simulink model "Crane3D_first_lqr"  (R2015a)
settings: Solver=ode5  SolverMode=SingleTasking  StartTime=0.0  StopTime=30  FixedStep=T0  RelTol=1e-3  AbsTol=1e-6
values from neighbouring files (symbols this model uses):
  Al = [0  1     0 0 ... (first row only)    [req_lqr.m]
  Bl = [0; Km/T; 0; K*Km*omega^2/T]    [req_lqr.m]
  Cl = [1 0 0 0 ... (first row only)    [req_lqr.m]
  Klqr = lqr(Al,Bl,Q,R)    [req_lqr.m]
  L = transpose(place(transpose(Al),transpose(Cl), [-11 -10 -9 -11]))    [req_lqr.m]
  X0 = [0 0 0 0]    [req_lqr.m]
undefined symbols (not defined in the file or in its folder): Crane3D_RangeBit, Crane3D_ScaleCoeff
undefined symbols (not defined in the file): RTDAC4PCIBaseAddress, T0
settings Model: SimulationMode=external  CovSFcnEnable=off  ExtModeTrigDuration=100000  Creator=jims  LastModifiedBy=Student
settings DataIOCC: ExternalInput=[]  InitialState=[]  LimitDataPoints=off  MaxDataPoints=5000  SignalLoggingSaveFormat=ModelDataLogs  SaveOutput=off  SaveTime=off
settings OptimizationCC: BooleanDataType=off  OptimizeBlockIOStorage=off  BufferReuse=off  GlobalBufferReuse=off  ExpressionFolding=off  ExpressionDepthLimit=2147483647  LocalBlockOutputs=off  InitFltsAndDblsToZero=on
settings DebuggingCC: SaveWithParameterizedLinksMsg=none  UnderspecifiedInitializationDetection=Classic  MergeDetectMultiDrivingBlocksExec=none  SignalResolutionControl=TryResolveAllWithWarning  MultiTaskDSMMsg=warning  MultiTaskCondExecSysMsg=none  IntegerOverflowMsg=none  FcnCallInpInsideContextMsg=UseLocalSettings  StateNameClashWarn=warning  IntegerSaturationMsg=none
settings HardwareCC: ProdBitPerLong=64  ProdBitPerPointer=64  ProdIntDivRoundTo=Zero  ProdEndianess=LittleEndian  ProdWordSize=64  ProdHWDeviceType=Intel->x86-64  TargetBitPerLong=64  TargetBitPerPointer=64  TargetIntDivRoundTo=Zero  TargetEndianess=LittleEndian  TargetWordSize=64  TargetHWDeviceType=Intel->x86-64
settings RTWCC: SystemTargetFile=rtwin.tlc  TemplateMakefile=rtwin.tmf  Description=Real-Time Windows Target
settings RTWinTargetCC: TargetFcnLib=ansi_tfl_tmw.mat  TargetPreCompLibLocation=C:\Program Files\MATLAB\R2015aSP1\toolbox\sldrt\lib\win64  ModelReferenceCompliant=off  CompOptLevelCompliant=off

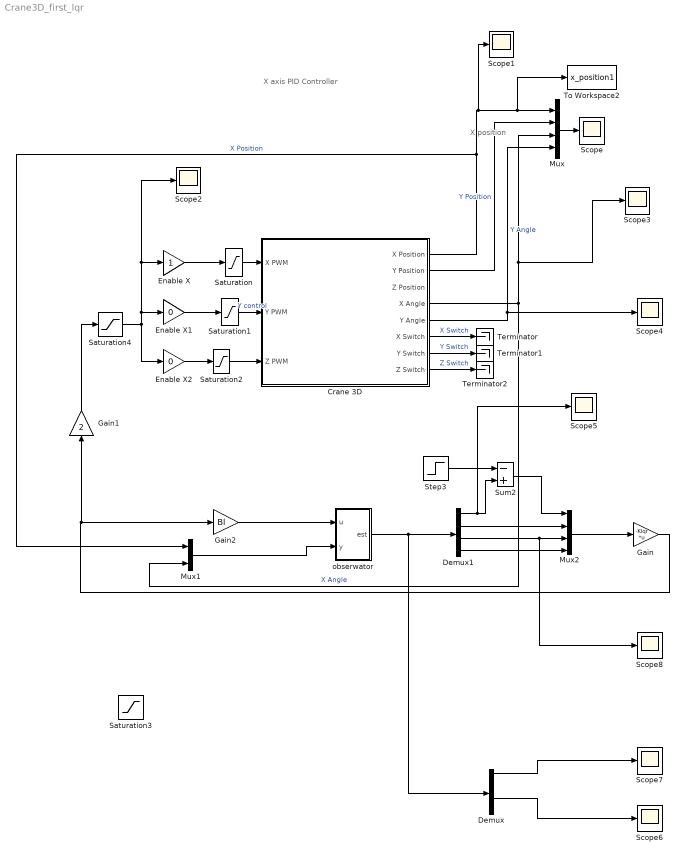
== system Crane3D_first_lqr ==
  note: X axis PID Controller
  note: X position
  Crane 3D : Subsystem  mask{BaseAddress=RTDAC4PCIBaseAddress, T0=T0}
      mask prompts: BaseAddress "Base Address:"; T0 "Sampling Period:"
      mask Display: image(imread('crane.jpeg'))
  Demux : Demux
  Demux1 : Demux
  Enable X : Gain  SaturateOnIntegerOverflow=on  OutDataTypeStr=Inherit: Same as input  ParamDataTypeStr=Inherit: Same as input
  Enable X1 : Gain  Gain=0  SaturateOnIntegerOverflow=on  OutDataTypeStr=Inherit: Same as input  ParamDataTypeStr=Inherit: Same as input
  Enable X2 : Gain  Gain=0  SaturateOnIntegerOverflow=on  OutDataTypeStr=Inherit: Same as input  ParamDataTypeStr=Inherit: Same as input
  Gain : Gain  Gain=-Klqr  Multiplication=Matrix(K*u) (u vector)
  Gain1 : Gain  Gain=2
  Gain2 : Gain  Gain=Bl
  Mux : Mux
  Mux1 : Mux  Inputs=2
  Mux2 : Mux
  Saturation{,1..4} (5 alike) : Saturate  UpperLimit=1  LowerLimit=-1
  Scope{,1..8} (9 alike) : Scope
      Scope settings: YMin=-0.25  YMax=4  SaveName=wsp
      Scope1 settings: YMin=1.38778e-17  YMax=0.35  SaveName=wsp1
      Scope2 settings: YMin=-0.1  YMax=0.65  SaveName=sterowanie
      Scope3 settings: YMin=-0.01  YMax=0.05  SaveName=wsp3
      Scope4 settings: YMin=-0.3  YMax=0.3  SaveName=wsp2
      Scope5 settings: YMin=0  YMax=0.12  SaveName=ScopeData2
      Scope6 settings: YMin=0.0881  YMax=0.088425
      Scope7 settings: YMin=0.27125  YMax=0.274
      Scope8 settings: YMin=-0.4  YMax=0.2  SaveName=ScopeData3
  Step3 : Step  Before=0.1  After=0.3  SampleTime=0
  Sum2 : Sum  Inputs=-+
  Terminator : Terminator
  Terminator1 : Terminator
  Terminator2 : Terminator
  To Workspace2 : ToWorkspace  VariableName=x_position1  SampleTime=-1
  "obserwator " : Subsystem
  wires:
  Crane 3D/6(X Switch) -> Terminator/1  "X Switch"
  Crane 3D/7(Y Switch) -> Terminator1/1  "Y Switch"
  Crane 3D/8(Z Switch) -> Terminator2/1  "Z Switch"
  Enable X/1 -> Saturation/1
  Crane 3D/4(X Angle) -> Mux/3, Scope3/1, Mux1/2  "X Angle"
  Crane 3D/5(Y Angle) -> Mux/4, Scope4/1  "Y Angle"
  Crane 3D/1(X Position) -> Mux1/1, Scope1/1, To Workspace2/1, Mux/1  "X Position"
  Saturation2/1 -> Crane 3D/3(Z PWM)
  Saturation1/1 -> Crane 3D/2(Y PWM)  "Y control"
  Saturation/1 -> Crane 3D/1(X PWM)
  Mux/1 -> Scope/1
  Crane 3D/2(Y Position) -> Mux/2  "Y Position"
  Enable X1/1 -> Saturation1/1
  Enable X2/1 -> Saturation2/1
  "obserwator "/1(est) -> Demux/1, Demux1/1
  Demux/3 -> Scope6/1
  Demux/1 -> Scope7/1
  Step3/1 -> Sum2/1
  Demux1/1 -> Scope5/1, Sum2/2
  Mux2/1 -> Gain/1
  Sum2/1 -> Mux2/1
  Demux1/2 -> Mux2/2
  Demux1/3 -> Scope8/1, Mux2/3
  Demux1/4 -> Mux2/4
  Saturation4/1 -> Enable X1/1, Scope2/1, Enable X/1, Enable X2/1
  Gain2/1 -> "obserwator "/1(u)
  Mux1/1 -> "obserwator "/2(y)
  Gain/1 -> Gain2/1, Gain1/1
  Gain1/1 -> Saturation4/1

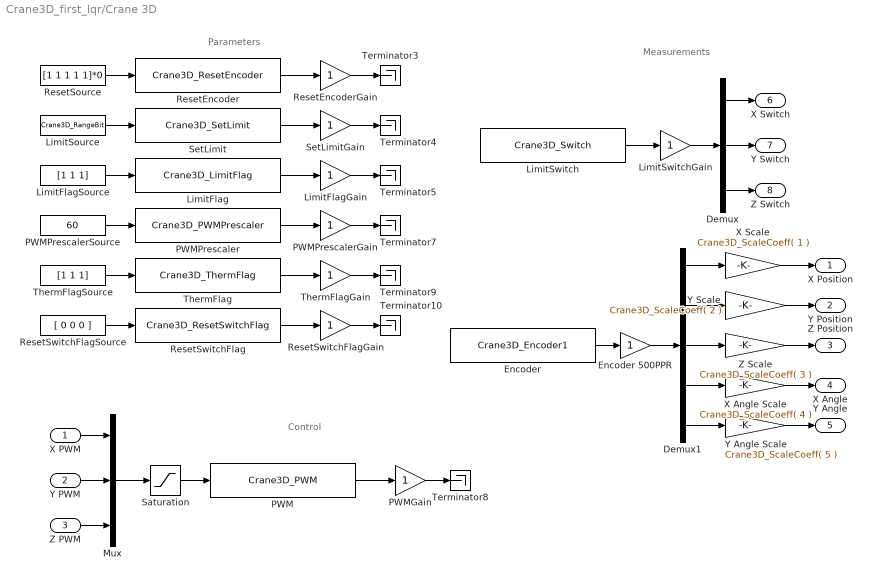
== system Crane3D_first_lqr/Crane 3D ==
  note: Parameters
  note: Control
  note: Measurements
  X PWM : Inport
  Y PWM : Inport  Port=2
  Z PWM : Inport  Port=3
  Demux : Demux  Outputs=3
  Demux1 : Demux  Outputs=5
  Encoder : S-Function  FunctionName=Crane3D_Encoder1  Parameters=BaseAddress, T0
  Encoder 500PPR : Gain  SaturateOnIntegerOverflow=on  OutDataTypeStr=Inherit: Same as input  ParamDataTypeStr=Inherit: Same as input
  LimitFlag : S-Function  FunctionName=Crane3D_LimitFlag  Parameters=BaseAddress, T0
  LimitFlagGain : Gain  SaturateOnIntegerOverflow=on  OutDataTypeStr=Inherit: Same as input  ParamDataTypeStr=Inherit: Same as input
  LimitFlagSource : Constant  Value=[1 1 1]
  LimitSource : Constant  Value=Crane3D_RangeBit
  LimitSwitch : S-Function  FunctionName=Crane3D_Switch  Parameters=BaseAddress, T0
  LimitSwitchGain : Gain  SaturateOnIntegerOverflow=on  OutDataTypeStr=Inherit: Same as input  ParamDataTypeStr=Inherit: Same as input
  Mux : Mux  Inputs=3
  PWM : S-Function  FunctionName=Crane3D_PWM  Parameters=BaseAddress, T0
  PWMGain : Gain  SaturateOnIntegerOverflow=on  OutDataTypeStr=Inherit: Same as input  ParamDataTypeStr=Inherit: Same as input
  PWMPrescaler : S-Function  FunctionName=Crane3D_PWMPrescaler  Parameters=BaseAddress, T0
  PWMPrescalerGain : Gain  SaturateOnIntegerOverflow=on  OutDataTypeStr=Inherit: Same as input  ParamDataTypeStr=Inherit: Same as input
  PWMPrescalerSource : Constant  Value=60
  ResetEncoder : S-Function  FunctionName=Crane3D_ResetEncoder  Parameters=BaseAddress, T0
  ResetEncoderGain : Gain  SaturateOnIntegerOverflow=on  OutDataTypeStr=Inherit: Same as input  ParamDataTypeStr=Inherit: Same as input
  ResetSource : Constant  Value=[1 1 1 1 1]*0
  "ResetSwitchFlag " : S-Function  FunctionName=Crane3D_ResetSwitchFlag  Parameters=BaseAddress, T0
  ResetSwitchFlagGain : Gain  SaturateOnIntegerOverflow=on  OutDataTypeStr=Inherit: Same as input  ParamDataTypeStr=Inherit: Same as input
  ResetSwitchFlagSource : Constant  Value=[ 0 0 0 ]
  Saturation : Saturate  UpperLimit=1  LowerLimit=-1
  SetLimit : S-Function  FunctionName=Crane3D_SetLimit  Parameters=BaseAddress, T0
  SetLimitGain : Gain  SaturateOnIntegerOverflow=on  OutDataTypeStr=Inherit: Same as input  ParamDataTypeStr=Inherit: Same as input
  Terminator{3..5,7..10} (7 alike) : Terminator
  "ThermFlag " : S-Function  FunctionName=Crane3D_ThermFlag  Parameters=BaseAddress, T0
  ThermFlagGain : Gain  SaturateOnIntegerOverflow=on  OutDataTypeStr=Inherit: Same as input  ParamDataTypeStr=Inherit: Same as input
  ThermFlagSource : Constant  Value=[1 1 1]
  X Angle Scale : Gain  Gain=Crane3D_ScaleCoeff( 4 )  OutDataTypeStr=Inherit: Same as input  ParamDataTypeStr=Inherit: Same as input
  X Scale : Gain  Gain=Crane3D_ScaleCoeff( 1 )  OutDataTypeStr=Inherit: Same as input  ParamDataTypeStr=Inherit: Same as input
  Y Angle Scale : Gain  Gain=Crane3D_ScaleCoeff( 5 )  OutDataTypeStr=Inherit: Same as input  ParamDataTypeStr=Inherit: Same as input
  Y Scale : Gain  Gain=Crane3D_ScaleCoeff( 2 )  OutDataTypeStr=Inherit: Same as input  ParamDataTypeStr=Inherit: Same as input
  Z Scale : Gain  Gain=Crane3D_ScaleCoeff( 3 )  OutDataTypeStr=Inherit: Same as input  ParamDataTypeStr=Inherit: Same as input
  X Position : Outport  InitialOutput=0
  Y Position : Outport  Port=2  InitialOutput=0
  Z Position : Outport  Port=3  InitialOutput=0
  X Angle : Outport  Port=4  InitialOutput=0
  Y Angle : Outport  Port=5  InitialOutput=0
  X Switch : Outport  Port=6  InitialOutput=0
  Y Switch : Outport  Port=7  InitialOutput=0
  Z Switch : Outport  Port=8  InitialOutput=0
  wires:
  Encoder 500PPR/1 -> Demux1/1
  Encoder/1 -> Encoder 500PPR/1
  Saturation/1 -> PWM/1
  Mux/1 -> Saturation/1
  PWM/1 -> PWMGain/1
  PWMGain/1 -> Terminator8/1
  ResetEncoder/1 -> ResetEncoderGain/1
  SetLimit/1 -> SetLimitGain/1
  LimitFlag/1 -> LimitFlagGain/1
  PWMPrescaler/1 -> PWMPrescalerGain/1
  "ThermFlag "/1 -> ThermFlagGain/1
  "ResetSwitchFlag "/1 -> ResetSwitchFlagGain/1
  ResetSource/1 -> ResetEncoder/1
  LimitSource/1 -> SetLimit/1
  LimitFlagSource/1 -> LimitFlag/1
  PWMPrescalerSource/1 -> PWMPrescaler/1
  ThermFlagSource/1 -> "ThermFlag "/1
  ResetSwitchFlagSource/1 -> "ResetSwitchFlag "/1
  ResetEncoderGain/1 -> Terminator3/1
  SetLimitGain/1 -> Terminator4/1
  LimitFlagGain/1 -> Terminator5/1
  PWMPrescalerGain/1 -> Terminator7/1
  ThermFlagGain/1 -> Terminator9/1
  ResetSwitchFlagGain/1 -> Terminator10/1
  Z PWM/1 -> Mux/3
  Y PWM/1 -> Mux/2
  X PWM/1 -> Mux/1
  LimitSwitch/1 -> LimitSwitchGain/1
  LimitSwitchGain/1 -> Demux/1
  Demux/1 -> X Switch/1
  Demux/2 -> Y Switch/1
  Demux/3 -> Z Switch/1
  Z Scale/1 -> Z Position/1
  X Scale/1 -> X Position/1
  Y Scale/1 -> Y Position/1
  Y Angle Scale/1 -> Y Angle/1
  X Angle Scale/1 -> X Angle/1
  Demux1/5 -> Y Angle Scale/1
  Demux1/4 -> X Angle Scale/1
  Demux1/3 -> Z Scale/1
  Demux1/2 -> Y Scale/1
  Demux1/1 -> X Scale/1

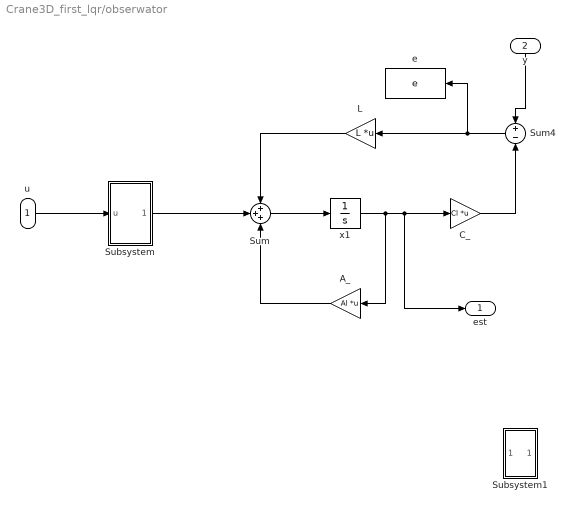
== system Crane3D_first_lqr/obserwator  ==
  u : Inport
  y : Inport  Port=2
  A_ : Gain  Gain=Al  Multiplication=Matrix(K*u) (u vector)
  C_ : Gain  Gain=Cl  Multiplication=Matrix(K*u) (u vector)
  L : Gain  Gain=L  Multiplication=Matrix(K*u) (u vector)
  Subsystem : Subsystem
  Subsystem1 : Subsystem
  Sum : Sum  Inputs=+++
  Sum4 : Sum  Inputs=+-
  e : ToWorkspace  VariableName=e  SaveFormat=Timeseries  SampleTime=-1
  x1 : Integrator  InitialCondition=X0
  est : Outport
  wires:
  y/1 -> Sum4/1
  L/1 -> Sum/1
  Sum/1 -> x1/1
  Sum4/1 -> e/1, L/1
  x1/1 -> A_/1, est/1, C_/1
  A_/1 -> Sum/3
  C_/1 -> Sum4/2
  u/1 -> Subsystem/1(u)
  Subsystem/1(Out1) -> Sum/2

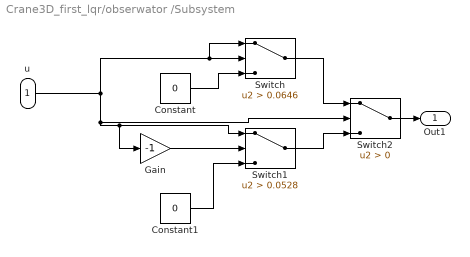
== system Crane3D_first_lqr/obserwator /Subsystem ==
  u : Inport
  Constant : Constant  Value=0
  Constant1 : Constant  Value=0
  Gain : Gain  Gain=-1
  Switch : Switch  Criteria=u2 > Threshold  Threshold=0.0646
  Switch1 : Switch  Criteria=u2 > Threshold  Threshold=0.0528
  Switch2 : Switch  Criteria=u2 > Threshold
  Out1 : Outport
  wires:
  Switch1/1 -> Switch2/3
  Gain/1 -> Switch1/2
  Constant/1 -> Switch/3
  u/1 -> Switch/1, Switch/2, Switch2/2, Gain/1, Switch1/1
  Switch/1 -> Switch2/1
  Switch2/1 -> Out1/1
  Constant1/1 -> Switch1/3

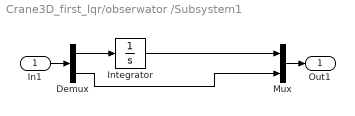
== system Crane3D_first_lqr/obserwator /Subsystem1 ==
  In1 : Inport
  Demux : Demux  Outputs=2
  Integrator : Integrator
  Mux : Mux  Inputs=2
  Out1 : Outport
  wires:
  Demux/1 -> Integrator/1
  In1/1 -> Demux/1
  Demux/2 -> Mux/2
  Mux/1 -> Out1/1
  Integrator/1 -> Mux/1
